simulink model "modeloLineal"  (R2022a)
settings: Solver=VariableStepAuto  StartTime=0.0  StopTime=100  FixedStep=0.148852529274642  RelTol=1e-3
model workspace (MAT data in the model file):
  ca = 0.02
  cb = 0.2
  ea = 0.06
  eb = 0.02
  pa = 6.5
  pb = 6.5
  u = 0.105
  v = 7.5
settings Model: Creator=Asus  LastModifiedBy=Abelino
settings DataIOCC: SaveFormat=Array  OutputTimes=tout

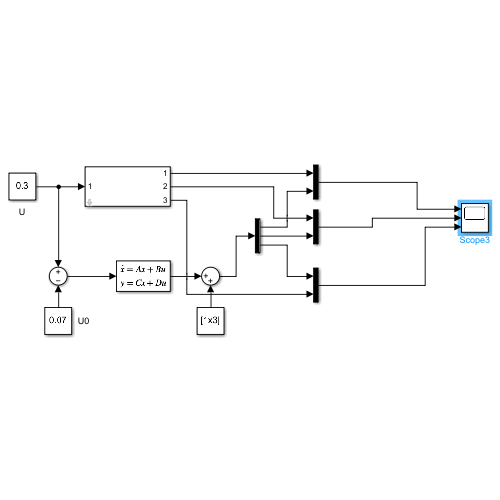
[thumbnail: Simulink's stored preview of the top-level diagram]
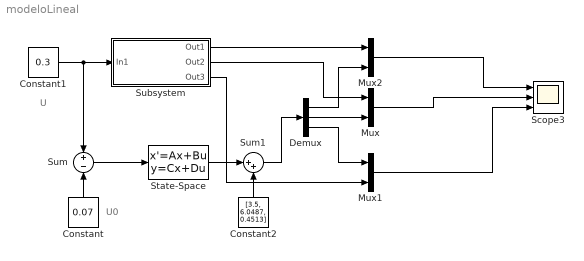
== system modeloLineal ==
  note: U0
  note: U
  Constant : Constant  Value=0.07
  Constant1 : Constant  Value=0.3
  Constant2 : Constant  Value=[3.5, 6.0487, 0.4513]
  Demux : Demux  Outputs=3
  Mux : Mux  Inputs=2
  Mux1 : Mux  Inputs=2
  Mux2 : Mux  Inputs=2
  Scope3 : Scope  NumInputPorts=3
  State-Space : StateSpace  A=[0, 0.07, 0.07; -0.121, 0.0003, 1.2097; 0.121, -0.0703, -1.2797]  B=[-3.5; 0; 3.5]  C=[1, 0, 0 ; 0, 1, 0; 0, 0, 1]  D=[0; 0; 0]  InitialCondition=[0,0,0]  AllowTunableDMatrix=on
  Subsystem : Subsystem  mask{ea=0.06, eb=0.02, ca=0.02, cb=0.2, pa=3, pb=3, v=4}
      mask prompts: ea "Tasa de extinción competidor A"; eb "Tasa de extinción del competidor B"; ca "Tasa de colonización del competidor A"; cb "Tasa de colonización del competidor B"; pa "Condición inicial x1"; pb "Condicion inicial x2"; v "Condicion inicial x3"
  Sum : Sum  Inputs=+-
  Sum1 : Sum  Inputs=|++
  wires:
  Subsystem/2(Out2) -> Mux/1
  Subsystem/3(Out3) -> Mux1/2
  Subsystem/1(Out1) -> Mux2/1
  Constant1/1 -> Subsystem/1(In1), Sum/1
  Sum/1 -> State-Space/1
  State-Space/1 -> Sum1/1
  Constant2/1 -> Sum1/2
  Sum1/1 -> Demux/1
  Demux/1 -> Mux2/2
  Demux/2 -> Mux/2
  Demux/3 -> Mux1/1
  Mux2/1 -> Scope3/1
  Mux/1 -> Scope3/2
  Mux1/1 -> Scope3/3
  Constant/1 -> Sum/2

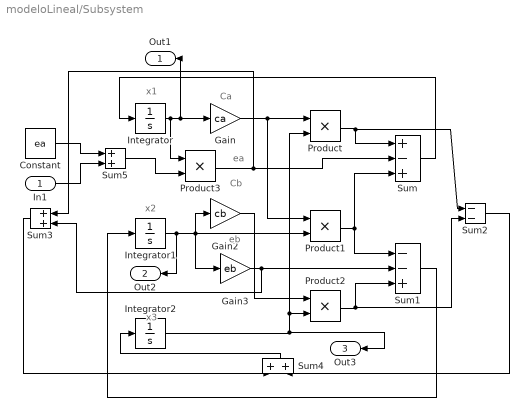
== system modeloLineal/Subsystem ==
  note: x1
  note: x3
  note: x2
  note: eb
  note: Cb
  note: ea
  note: Ca
  In1 : Inport
  Constant : Constant  Value=ea
  Gain : Gain  Gain=ca
  Gain2 : Gain  Gain=cb
  Gain3 : Gain  Gain=eb
  Integrator : Integrator  InitialCondition=pa  LimitOutput=on  LowerSaturationLimit=0
  Integrator1 : Integrator  InitialCondition=pb  LimitOutput=on  LowerSaturationLimit=0
  Integrator2 : Integrator  InitialCondition=v  LimitOutput=on  LowerSaturationLimit=0
  Product{,1..3} (4 alike) : Product
  Sum : Sum  Inputs=+-+
  Sum1 : Sum  Inputs=--+
  Sum2 : Sum  Inputs=--
  Sum3 : Sum
  Sum4 : Sum
  Sum5 : Sum
  Out1 : Outport
  Out2 : Outport  Port=2
  Out3 : Outport  Port=3
  wires:
  Integrator/1 -> Gain/1, Out1/1, Product3/1
  Gain/1 -> Product1/1, Product/1
  Integrator2/1 -> Product/2, Product2/2, Out3/1
  Sum4/1 -> Integrator2/1
  Product2/1 -> Sum2/2, Sum1/3
  Sum2/1 -> Sum4/2
  Product/1 -> Sum2/1, Sum/1
  Gain2/1 -> Product2/1
  Gain3/1 -> Sum3/2, Sum1/2
  Sum3/1 -> Sum4/1
  Integrator1/1 -> Out2/1, Gain3/1, Gain2/1, Product1/2
  Sum/1 -> Integrator/1
  Product1/1 -> Sum/3, Sum1/1
  Sum1/1 -> Integrator1/1
  Product3/1 -> Sum3/1, Sum/2
  Constant/1 -> Sum5/1
  In1/1 -> Sum5/2
  Sum5/1 -> Product3/2
